simulink model "PVarray"  (R2020a)
settings: Solver=VariableStepAuto  StartTime=0.0  StopTime=.05  RelTol=1e-3
libraries: powerlib x2, re_lib x1
settings Model: Creator=hp  LastModifiedBy=hp

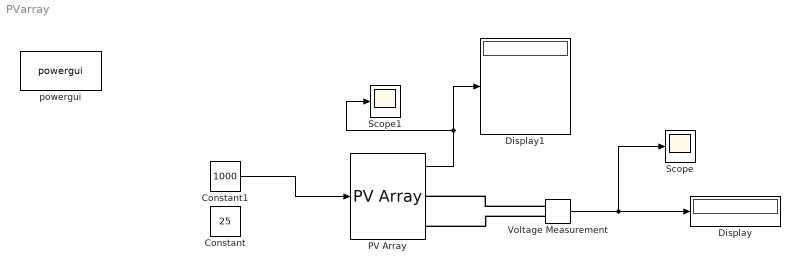
== system PVarray ==
  Constant : Constant  Value=25
  Constant1 : Constant  Value=1000
  Display : Display
  Display1 : Display
  PV Array : re_lib/Solar/PV Array  Npar=1  Nser=1  PlotType=array @ 1000 W/m2 & specified temperatures  S_vec="[ 1000  500  100 ]"  Temp_C_vec="[ 45 25  ]"  ModuleName=Bosch Solar Energy c-Si M 60 NA30117 230W  PlotWhenSelected=off  Pm=234.63  Ncell=60  Voc=37  Isc=8.4  Vm=29.7  Im=7.9  beta_Voc_pc=-0.366  alpha_Isc_pc=0.099  beta_Voc=-0.13542  alpha_Isc=0.008316  IL=8.428  I0=3.7086e-10  nI=1.007  Rsh=370.6909  Rs=0.35119  RobustModel=on  RobustCellTemperature=25  BAL=on  Tc=1e-6  Tfilter=5e-5
  Scope : Scope
  Scope1 : Scope
  Voltage Measurement : powerlib/Measurements/Voltage Measurement  PhasorSimulation=off  OutputType=Complex  PSBequivalent=0
  powergui : powerlib/powergui  Priority=1  SimulationMode=Discrete  SampleTime=50e-6  frequency=60  Iterations=50  frequencyindice=0  Pbase=100e6  ErrMax=1e-4  UnitsV=kV  UnitsW=MW  buscounter=0  FunctionMessages=off  echomessages=off  EnableUseOfTLC=off  CurrentSourceSwitches=off  DisableSnubberDevices=off  DisableRonSwitches=off  DisableVfSwitches=off  DisplayEquations=off  AutomaticDiscreteSolvers=off  SolverType=Tustin/Backward Euler (TBE)  Interpol=off  ExternalGateDelay=off  methode=off  Ts=100  x0status=blocks  SPID=on  SwTol=0  HookPort=off  NonlinearTolerance=1e-4  nMaxIteration=100  ContinueOnMaxIteration=off  RestoreLinks=warning  ResistiveCurrentMeasurement=off  Frange=[0:2:500]  Ylog=off  Xlog=on  ShowGrid=off  save=off  variable=ZData  structure=0  ZoomFFT=off  StartTime=0.0  cycles=1  DisplayStyle=1  fundamental=60  FreqAxis=off  MaxFrequency=1000  frequencyindicesteady=1  RmsSteady=1  display=off
  wires:
  Constant1/1 -> PV Array/1
  Voltage Measurement/1 -> Scope/1, Display/1
  PV Array/1 -> Scope1/1, Display1/1
  connections:
  Voltage Measurement/LConn1 -- PV Array/RConn1
  Voltage Measurement/LConn2 -- PV Array/RConn2
